simulink model "ej2slx"  (R2020a)
settings: Solver=VariableStepAuto  StartTime=0.0  StopTime=100  RelTol=1e-3
values from neighbouring files (symbols this model uses):
  messi = SerialLink([links{:}], 'tool', Tool, 'name', 'messi')    [Ej_01.m]    (also in Ej_02.m)
undefined symbols (not defined in the file or in its folder): slcoulomb
libraries: roblocks x13
settings Model: Creator=mpier  LastModifiedBy=mpier

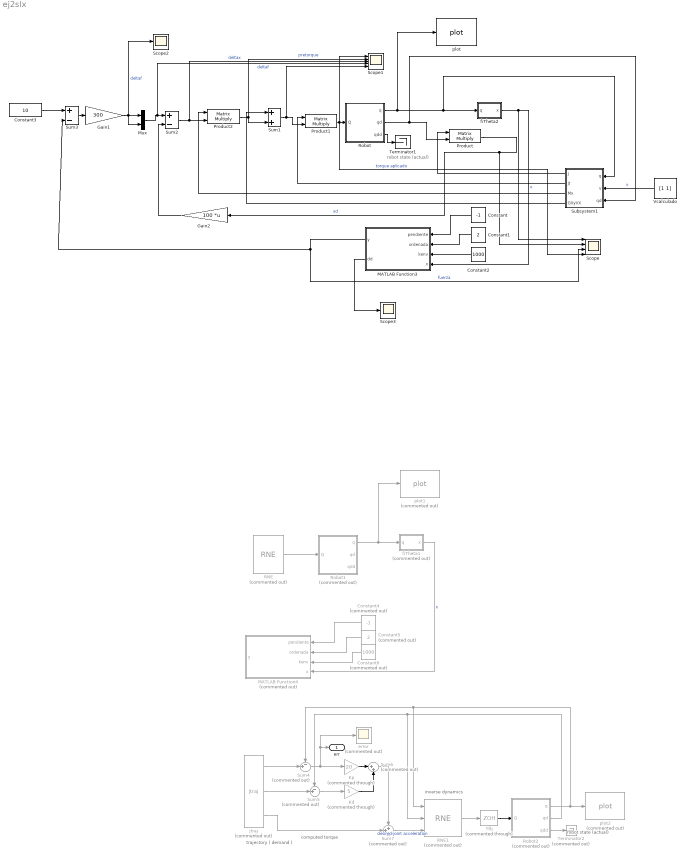
== system ej2slx ==
  note: robot state
      | (actual)
  note: computed torque
  note: trajectory
      | ( demand )
  note: inverse dynamics
  note: robot state
      | (actual)
  Constant : Constant  Value=-1
  Constant1 : Constant  Value=2
  Constant2 : Constant  Value=1000
  Constant3 : Constant  Value=10
  Constant4 : Constant  Commented=on  Value=-1
  Constant5 : Constant  Commented=on  Value=2
  Constant6 : Constant  Commented=on  Value=1000
  Gain1 : Gain  Gain=300
  Gain2 : Gain  Gain=100  Multiplication=Matrix(K*u)
  Kd : Gain  Commented=through  Gain=5  SaturateOnIntegerOverflow=on  OutDataTypeStr=Inherit: Same as input  ParamDataTypeStr=Inherit: Same as input
  Kp : Gain  Commented=through  Gain=20  SaturateOnIntegerOverflow=on  OutDataTypeStr=Inherit: Same as input  ParamDataTypeStr=Inherit: Same as input
  MATLAB Function3 : MATLAB Function  TreatAsAtomicUnit=on
  MATLAB Function4 : MATLAB Function  Commented=on  TreatAsAtomicUnit=on
  Mux : Mux  Inputs=2
  Product : Product  Multiplication=Matrix(*)
  Product1 : Product  Multiplication=Matrix(*)
  Product2 : Product  Multiplication=Matrix(*)
  RNE : roblocks/Arm/RNE  Commented=on  robot=messi  grav=[0 0 9.81]
  RNE1 : roblocks/Arm/RNE  Commented=on  robot=messi  grav=[0 0 9.81]
  Robot : Subsystem  AncestorBlock=roblocks/Arm/Robot  mask{robot=messi, q0=[-20.53*pi/180  pi/4+abs(-20.53*pi/180)]}
      mask prompts: robot "Robot object"; q0 "Initial state"
      mask help: Rigid-body dynamic model of robot.
      mask init:
      | if isa(robot, 'SerialLink')
      |     rname = robot.name;
      |     %fprintf('**robot name is %s\n', rname);
      | else
      |     rname = '';
      |     n = 0
      | end
      mask Help:
      | Simulates the forward (direct) rigid-body dynamics of the robot described
      | by the given robot object.  For given applied joint torque/force it computes
      | the instaneous joint coordinates, velocities and acclerations.
      | 
      | 
      | <b>Parameters::</b>
      | 
      | robot (SerialLink) a dynamic model of an N-link serial link manipulator
      | q0 (1xN)  Initial joint coordinates
      | 
      | <b>Inputs::</b>
      | 
      | Q (1xN) the generalized joint force (torque or force) required to achieve
      | the motion state (q, qd, qdd).
      | 
      | <b>Outputs::</b>
      | 
      | q (1xN) joint coordinates
      | qd (1xN) joint coordinate velocity
      | qdd (1xN) joint coordinate acceleration
      | 
      | 
      | <b>Notes::</b>
      | 
      | - Required to simulate robot rigid body motion.
      | - Implemented using the recursive Newton-Euler scheme (RNE).
      | - A wrapper for the Toolbox method accel() which in turn depends on the
      |   method rne().
      mask Display:
      | port_label('input', 1, 'Q')
      | port_label('output', 1, 'q')
      | port_label('output', 2, 'qd')
      | port_label('output', 3, 'qdd')
      | text(0.1, 0.9,  rname, 'horizontalAlignment', 'left')
  Robot1 : Subsystem  Commented=on  AncestorBlock=roblocks/Arm/Robot  mask{robot=messi, q0=[0 0]}
      mask prompts: robot "Robot object"; q0 "Initial state"
      mask help: Rigid-body dynamic model of robot.
      mask init:
      | if isa(robot, 'SerialLink')
      |     rname = robot.name;
      |     %fprintf('**robot name is %s\n', rname);
      | else
      |     rname = '';
      |     n = 0
      | end
      mask Help:
      | Simulates the forward (direct) rigid-body dynamics of the robot described
      | by the given robot object.  For given applied joint torque/force it computes
      | the instaneous joint coordinates, velocities and acclerations.
      | 
      | 
      | <b>Parameters::</b>
      | 
      | robot (SerialLink) a dynamic model of an N-link serial link manipulator
      | q0 (1xN)  Initial joint coordinates
      | 
      | <b>Inputs::</b>
      | 
      | Q (1xN) the generalized joint force (torque or force) required to achieve
      | the motion state (q, qd, qdd).
      | 
      | <b>Outputs::</b>
      | 
      | q (1xN) joint coordinates
      | qd (1xN) joint coordinate velocity
      | qdd (1xN) joint coordinate acceleration
      | 
      | 
      | <b>Notes::</b>
      | 
      | - Required to simulate robot rigid body motion.
      | - Implemented using the recursive Newton-Euler scheme (RNE).
      | - A wrapper for the Toolbox method accel() which in turn depends on the
      |   method rne().
      mask Display:
      | port_label('input', 1, 'Q')
      | port_label('output', 1, 'q')
      | port_label('output', 2, 'qd')
      | port_label('output', 3, 'qdd')
      | text(0.1, 0.9,  rname, 'horizontalAlignment', 'left')
  Robot2 : Subsystem  Commented=on  AncestorBlock=roblocks/Arm/Robot  mask{robot=messi, q0=[0 0]}
      mask prompts: robot "Robot object"; q0 "Initial state"
      mask help: Rigid-body dynamic model of robot.
      mask init:
      | if isa(robot, 'SerialLink')
      |     rname = robot.name;
      |     %fprintf('**robot name is %s\n', rname);
      | else
      |     rname = '';
      |     n = 0
      | end
      mask Help:
      | Simulates the forward (direct) rigid-body dynamics of the robot described
      | by the given robot object.  For given applied joint torque/force it computes
      | the instaneous joint coordinates, velocities and acclerations.
      | 
      | 
      | <b>Parameters::</b>
      | 
      | robot (SerialLink) a dynamic model of an N-link serial link manipulator
      | q0 (1xN)  Initial joint coordinates
      | 
      | <b>Inputs::</b>
      | 
      | Q (1xN) the generalized joint force (torque or force) required to achieve
      | the motion state (q, qd, qdd).
      | 
      | <b>Outputs::</b>
      | 
      | q (1xN) joint coordinates
      | qd (1xN) joint coordinate velocity
      | qdd (1xN) joint coordinate acceleration
      | 
      | 
      | <b>Notes::</b>
      | 
      | - Required to simulate robot rigid body motion.
      | - Implemented using the recursive Newton-Euler scheme (RNE).
      | - A wrapper for the Toolbox method accel() which in turn depends on the
      |   method rne().
      mask Display:
      | port_label('input', 1, 'Q')
      | port_label('output', 1, 'q')
      | port_label('output', 2, 'qd')
      | port_label('output', 3, 'qdd')
      | text(0.1, 0.9,  rname, 'horizontalAlignment', 'left')
  Scope : Scope  NumInputPorts=4
  Scope1 : Scope  NumInputPorts=5
  Scope2 : Scope
  Scope3 : Scope
  Subsystem1 : Subsystem
  Sum1 : Sum
  Sum2 : Sum  Inputs=+-
  Sum3 : Sum  Inputs=+-
  Sum4 : Sum  Commented=on  Inputs=-+|  InputSameDT=on  SaturateOnIntegerOverflow=on  OutDataTypeStr=Inherit: Same as first input
  Sum5 : Sum  Commented=on  Inputs=-+|  InputSameDT=on  SaturateOnIntegerOverflow=on  OutDataTypeStr=Inherit: Same as first input
  Sum6 : Sum  Commented=on  Inputs=|++  InputSameDT=on  SaturateOnIntegerOverflow=on  OutDataTypeStr=Inherit: Same as first input
  Sum7 : Sum  Commented=on  Inputs=++|  InputSameDT=on  SaturateOnIntegerOverflow=on  OutDataTypeStr=Inherit: Same as first input
  Terminator1 : Terminator
  Terminator2 : Terminator  Commented=on
  Tfb : ZeroOrderHold  Commented=through  SampleTime=0.005
  Vcalculado : Constant  Value=[1 1]
  error : Scope  Commented=on
  fiTheta1 : Subsystem  Commented=on
  fiTheta2 : Subsystem
  jtraj : roblocks/Toolbox/jtraj  Commented=on  q0=q1  qf=q2  tmax=5  ts=-1
  plot : roblocks/Arm/plot  robot=messi  fps=10  holdplot=on
  plot1 : roblocks/Arm/plot  Commented=on  robot=messi  fps=10  holdplot=on
  plot2 : roblocks/Arm/plot  Commented=on  robot=messi  fps=10  holdplot=on
  err : Outport  VectorParamsAs1DForOutWhenUnconnected=off
  wires:
  Robot/3(qdd) -> Terminator1/1
  Subsystem1/4(GXyVX) -> Sum1/1
  Sum1/1 -> Scope1/5, Product1/2
  Product2/1 -> Scope1/2, Sum1/2  "pretorque"
  Constant/1 -> MATLAB Function3/1(pendiente)
  Constant1/1 -> MATLAB Function3/2(ordenada)
  Constant2/1 -> MATLAB Function3/3(kenv)
  Sum2/1 -> Scope1/3, Product2/2  "deltax"
  Sum3/1 -> Gain1/1
  MATLAB Function3/1(y) -> Scope/3, Sum3/2  "fuerza"
  RNE/1 -> Robot1/1(Q)
  Constant4/1 -> MATLAB Function4/1(pendiente)
  Constant5/1 -> MATLAB Function4/2(ordenada)
  Constant6/1 -> MATLAB Function4/3(kenv)
  Robot1/1(q) -> fiTheta1/1(q), plot1/1
  fiTheta1/1(x) -> MATLAB Function4/4(x)  "x"
  Sum6/1 -> Sum7/1
  jtraj/3 -> Sum7/2
  Sum4/1 -> error/1, err/1, Kp/1
  Tfb/1 -> Robot2/1(Q)
  Sum7/1 -> RNE1/3  "desired joint acceleration"
  Robot2/1(q) -> RNE1/1, Sum4/1, plot2/1
  Kp/1 -> Sum6/1
  Robot2/3(qdd) -> Terminator2/1
  Kd/1 -> Sum6/2
  Sum5/1 -> Kd/1
  RNE1/1 -> Tfb/1
  jtraj/1 -> Sum4/2
  jtraj/2 -> Sum5/2
  Robot2/2(qd) -> RNE1/2, Sum5/1
  Vcalculado/1 -> Subsystem1/2(v)  "v"
  Robot/1(q) -> plot/1, Subsystem1/1(q), fiTheta2/1(q)
  Robot/2(qd) -> Product/2, Subsystem1/3(qd)
  Product/1 -> Scope/2, Gain2/1  "xd"
  fiTheta2/1(x) -> Scope/1, MATLAB Function3/4(x)  "x"
  Subsystem1/2(jt) -> Product1/1
  Gain2/1 -> Sum2/2
  Constant3/1 -> Sum3/1
  Subsystem1/1(j) -> Product/1
  Product1/1 -> Scope1/1, Scope/4, Robot/1(Q)  "torque aplicado"
  Subsystem1/3(Mx) -> Product2/1
  Gain1/1 -> Scope2/1, Mux/2, Mux/1  "deltaf"
  Mux/1 -> Scope1/4, Sum2/1  "deltaf"
  MATLAB Function3/2(dd) -> Scope3/1

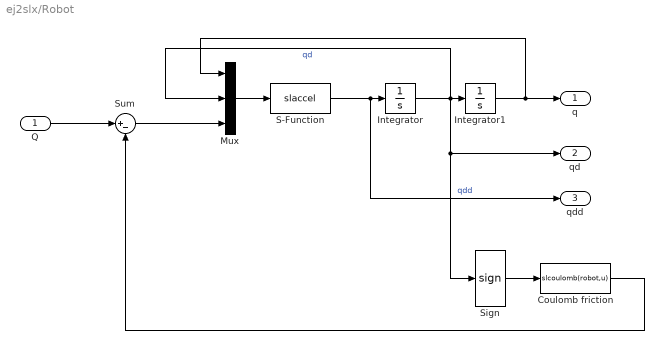
== system ej2slx/Robot ==
  Q : Inport
  Coulomb friction : MATLABFcn  MATLABFcn=slcoulomb(robot,u)  OutputDimensions=[robot.n 1]  Output1D=off
  Integrator : Integrator
  Integrator1 : Integrator  InitialCondition=q0
  Mux : Mux  Inputs=3
  S-Function : S-Function  FunctionName=slaccel  Parameters=robot  SFunctionDeploymentMode=off  EnableBusSupport=off
  Sign : Signum
  Sum : Sum  Inputs=|+-
  q : Outport  VectorParamsAs1DForOutWhenUnconnected=off
  qd : Outport  Port=2  VectorParamsAs1DForOutWhenUnconnected=off
  qdd : Outport  Port=3  VectorParamsAs1DForOutWhenUnconnected=off
  wires:
  S-Function/1 -> qdd/1, Integrator/1  "qdd"
  Mux/1 -> S-Function/1
  Integrator/1 -> Sign/1, qd/1, Integrator1/1, Mux/2  "qd"
  Integrator1/1 -> q/1, Mux/1
  Q/1 -> Sum/1
  Sum/1 -> Mux/3
  Coulomb friction/1 -> Sum/2
  Sign/1 -> Coulomb friction/1

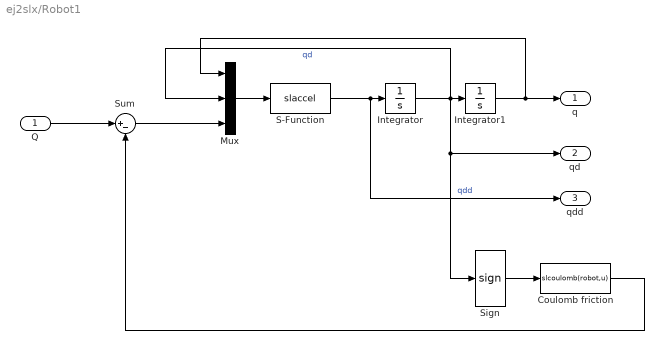
== system ej2slx/Robot1 ==
  Q : Inport
  Coulomb friction : MATLABFcn  MATLABFcn=slcoulomb(robot,u)  OutputDimensions=[robot.n 1]  Output1D=off
  Integrator : Integrator
  Integrator1 : Integrator  InitialCondition=q0
  Mux : Mux  Inputs=3
  S-Function : S-Function  FunctionName=slaccel  Parameters=robot  SFunctionDeploymentMode=off  EnableBusSupport=off
  Sign : Signum
  Sum : Sum  Inputs=|+-
  q : Outport  VectorParamsAs1DForOutWhenUnconnected=off
  qd : Outport  Port=2  VectorParamsAs1DForOutWhenUnconnected=off
  qdd : Outport  Port=3  VectorParamsAs1DForOutWhenUnconnected=off
  wires:
  S-Function/1 -> qdd/1, Integrator/1  "qdd"
  Mux/1 -> S-Function/1
  Integrator/1 -> Sign/1, qd/1, Integrator1/1, Mux/2  "qd"
  Integrator1/1 -> q/1, Mux/1
  Q/1 -> Sum/1
  Sum/1 -> Mux/3
  Coulomb friction/1 -> Sum/2
  Sign/1 -> Coulomb friction/1

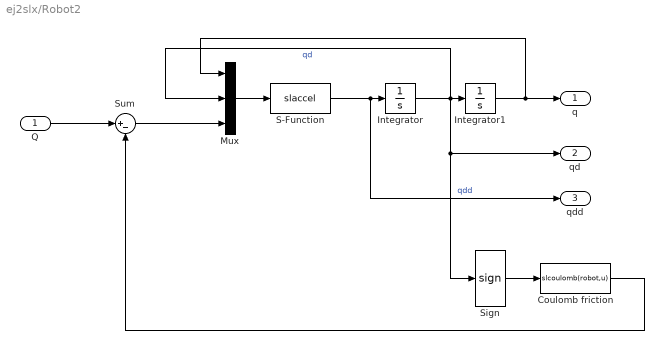
== system ej2slx/Robot2 ==
  Q : Inport
  Coulomb friction : MATLABFcn  MATLABFcn=slcoulomb(robot,u)  OutputDimensions=[robot.n 1]  Output1D=off
  Integrator : Integrator
  Integrator1 : Integrator  InitialCondition=q0
  Mux : Mux  Inputs=3
  S-Function : S-Function  FunctionName=slaccel  Parameters=robot  SFunctionDeploymentMode=off  EnableBusSupport=off
  Sign : Signum
  Sum : Sum  Inputs=|+-
  q : Outport  VectorParamsAs1DForOutWhenUnconnected=off
  qd : Outport  Port=2  VectorParamsAs1DForOutWhenUnconnected=off
  qdd : Outport  Port=3  VectorParamsAs1DForOutWhenUnconnected=off
  wires:
  S-Function/1 -> qdd/1, Integrator/1  "qdd"
  Mux/1 -> S-Function/1
  Integrator/1 -> Sign/1, qd/1, Integrator1/1, Mux/2  "qd"
  Integrator1/1 -> q/1, Mux/1
  Q/1 -> Sum/1
  Sum/1 -> Mux/3
  Coulomb friction/1 -> Sum/2
  Sign/1 -> Coulomb friction/1

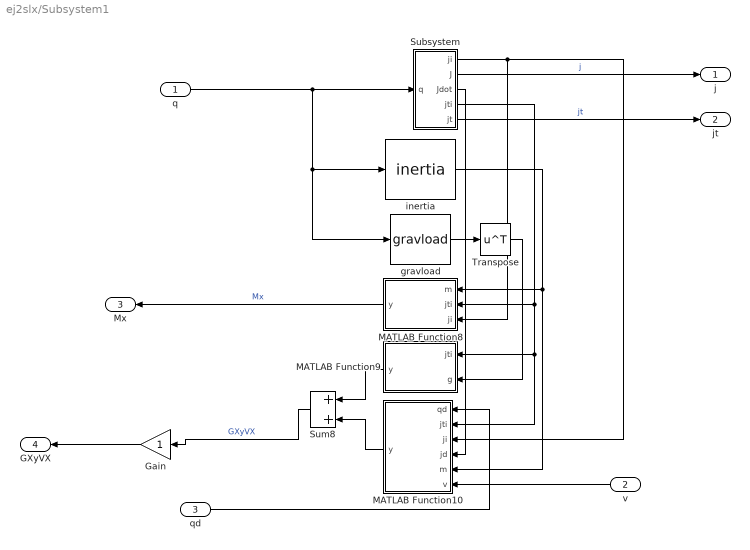
== system ej2slx/Subsystem1 ==
  q : Inport
  v : Inport  Port=2
  qd : Inport  Port=3
  Gain : Gain
  MATLAB Function10 : MATLAB Function  TreatAsAtomicUnit=on
  MATLAB Function8 : MATLAB Function  TreatAsAtomicUnit=on
  MATLAB Function9 : MATLAB Function  TreatAsAtomicUnit=on
  Subsystem : Subsystem
  Sum8 : Sum
  Transpose : Math  Operator=transpose  SaturateOnIntegerOverflow=on
  gravload : roblocks/Arm/gravload  robot=messi
  inertia : roblocks/Arm/inertia  robot=messi
  j : Outport
  jt : Outport  Port=2
  Mx : Outport  Port=3
  GXyVX : Outport  Port=4
  wires:
  Subsystem/1(ji) -> MATLAB Function8/3(ji), MATLAB Function10/3(ji)
  q/1 -> gravload/1, inertia/1, Subsystem/1(q)
  Subsystem/4(jti) -> MATLAB Function8/2(jti), MATLAB Function9/1(jti), MATLAB Function10/2(jti)
  MATLAB Function9/1(y) -> Sum8/1
  Sum8/1 -> Gain/1  "GXyVX"
  Subsystem/3(Jdot) -> MATLAB Function10/4(jd)
  MATLAB Function10/1(y) -> Sum8/2
  Subsystem/5(jt) -> jt/1  "jt"
  Subsystem/2(J) -> j/1  "j"
  qd/1 -> MATLAB Function10/1(qd)
  MATLAB Function8/1(y) -> Mx/1  "Mx"
  gravload/1 -> Transpose/1
  Transpose/1 -> MATLAB Function9/2(g)
  v/1 -> MATLAB Function10/6(v)
  Gain/1 -> GXyVX/1
  inertia/1 -> MATLAB Function10/5(m), MATLAB Function8/1(m)

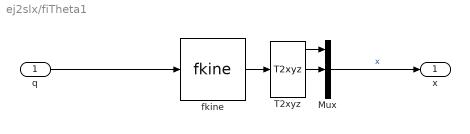
== system ej2slx/fiTheta1 ==
  q : Inport
  Mux : Mux  Inputs=3
  T2xyz : roblocks/Toolbox/T2xyz
  fkine : roblocks/Arm/fkine  robot=messi
  x : Outport
  wires:
  Mux/1 -> x/1  "x"
  fkine/1 -> T2xyz/1
  q/1 -> fkine/1
  T2xyz/2 -> Mux/2
  T2xyz/1 -> Mux/1

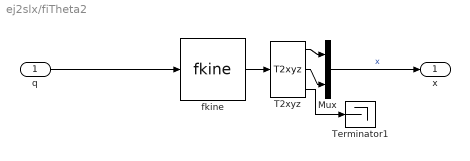
== system ej2slx/fiTheta2 ==
  q : Inport
  Mux : Mux  Inputs=2
  T2xyz : roblocks/Toolbox/T2xyz
  Terminator1 : Terminator
  fkine : roblocks/Arm/fkine  robot=messi
  x : Outport
  wires:
  Mux/1 -> x/1  "x"
  fkine/1 -> T2xyz/1
  q/1 -> fkine/1
  T2xyz/2 -> Mux/2
  T2xyz/1 -> Mux/1
  T2xyz/3 -> Terminator1/1

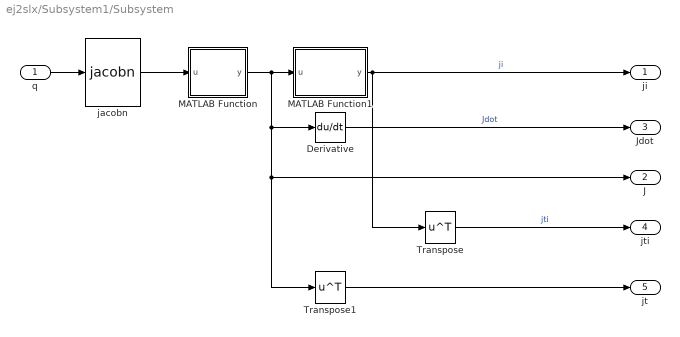
== system ej2slx/Subsystem1/Subsystem ==
  q : Inport
  Derivative : Derivative
  MATLAB Function : MATLAB Function  TreatAsAtomicUnit=on
  MATLAB Function1 : MATLAB Function  TreatAsAtomicUnit=on
  Transpose : Math  Operator=transpose  SaturateOnIntegerOverflow=on
  Transpose1 : Math  Operator=transpose  SaturateOnIntegerOverflow=on
  jacobn : roblocks/Arm/jacobn  robot=messi
  ji : Outport
  J : Outport  Port=2
  Jdot : Outport  Port=3
  jti : Outport  Port=4
  jt : Outport  Port=5
  wires:
  MATLAB Function1/1(y) -> Transpose/1, ji/1  "ji"
  Transpose/1 -> jti/1  "jti"
  q/1 -> jacobn/1
  Derivative/1 -> Jdot/1  "Jdot"
  Transpose1/1 -> jt/1
  jacobn/1 -> MATLAB Function/1(u)
  MATLAB Function/1(y) -> MATLAB Function1/1(u), J/1, Transpose1/1, Derivative/1

== matlab function ej2slx/Subsystem1/Subsystem/MATLAB Function1 ==
  data: u input; y output
function y = inversJac(u)

y = u^(-1);

== matlab function ej2slx/Subsystem1/Subsystem/MATLAB Function ==
  data: u input; y output
function y = extract(u)

y = u(1:2,1:2);

== matlab function ej2slx/MATLAB Function3 ==
  data: pendiente input; y output; ordenada input; kenv input; x input; dd output
function [y,dd] = ModeloFuerza(pendiente,ordenada,kenv,x)
d=abs(pendiente*x(1)-x(2)+ordenada)/sqrt((pendiente^2) +1);
yprima=x(1)*pendiente+ordenada;
if(yprima>x(2))
    d=0;
end
if((x(1)<0)||(x(2)<0))
    d=0;
end
temp=d*kenv;%*sqrt(2)/2;
dd=d;
y = temp;

== matlab function ej2slx/MATLAB Function4 ==
  data: pendiente input; y output; ordenada input; kenv input; x input
function y = ModeloFuerza(pendiente,ordenada,kenv,x)
d=abs(pendiente*x(1)-x(2)+ordenada)/sqrt((pendiente^2) +1);
yprima=x(1)*pendiente+ordenada;
if(yprima>x(2))
    d=0;
end
if((x(1)<0)||(x(2)<0))
    d=0;
end
temp=d*kenv*sqrt(2)/2;
y = [temp temp];

== matlab function ej2slx/Subsystem1/MATLAB Function8 ==
  data: m input; y output; jti input; ji input
function y = Mx(m,jti,ji)

y = jti*m*ji;

== matlab function ej2slx/Subsystem1/MATLAB Function9 ==
  data: jti input; y output; g input
function y = Gx(jti,g)

y = jti*g;

== matlab function ej2slx/Subsystem1/MATLAB Function10 ==
  data: qd input; y output; jti input; ji input; jd input; m input; v input
function y = Vx(qd,jti,ji,jd,m,v)

y = jti*(v-m*ji*jd*qd);
